simulink model "WindFarm_2023_BaseModel_v2"  (R2019a)
settings: Solver=ode1  StartTime=0.0  StopTime=2  FixedStep=Ts_Power  RelTol=1e-3
PostLoadFcn:
  | %% Init for wind PnO models - global system parameters
  | OVERRIDE_SSN_MEMORY_LIMIT=1;
  | Ts=50e-6;
  | % Ts=50e-10;
  | Ts_Power=Ts;
  | Ts_Control=2*Ts;
  | freq = 50;
  | Fnom=freq;
  | Vac=400e3;
InitFcn:
  | %% Init for wind PnO models - global system parameters
  | OVERRIDE_SSN_MEMORY_LIMIT=1;
  | Ts=50e-6;
  | % Ts=50e-10;
  | Ts_Power=Ts;
  | Ts_Control=2*Ts;
  | freq = 50;
  | Fnom=freq;
  | Vac=220e3;
values from neighbouring files (symbols this model uses):
  C0_Le_1 = C1_Le_1    (= 4.2e-07)    [windfarm_params.m]
  C0_Le_2 = C1_Le_2    (= 4.2e-07)    [windfarm_params.m]
  C0_Le_ON = 0.0084e-6    (= 8.4e-09)    [windfarm_params.m]
  C1_Le_1 = 0.42e-6    (= 4.2e-07)    [windfarm_params.m]
  C1_Le_2 = 0.42e-6    (= 4.2e-07)    [windfarm_params.m]
  C1_Le_ON = 0.0137e-6    (= 1.37e-08)    [windfarm_params.m]
  L0_fLA38a = X0_fLA38a / w    (= 0.00210440713644)    [windfarm_params.m]
  L0_fLB1 = X0_fLB1 / w    (= 0.00146508173004)    [windfarm_params.m]
  L0_fLB2 = X0_fLB2 / w    (= 0.00124721491041)    [windfarm_params.m]
  L0_Le_1 = X0_Le_1 / w    (= 0.00116978883173)    [windfarm_params.m]
  L0_Le_2 = X0_Le_2 / w    (= 0.00116978883173)    [windfarm_params.m]
  L0_Le_ON = 3.1544e-3    (= 0.0031544)    [windfarm_params.m]
  L1_fLA38a = X1_fLA38a / w    (= 0.00070146904548)    [windfarm_params.m]
  L1_fLB1 = X1_fLB1 / w    (= 0.00048836057668)    [windfarm_params.m]
  L1_fLB2 = X1_fLB2 / w    (= 0.000415738303471)    [windfarm_params.m]
  L1_Le_1 = X1_Le_1 / w    (= 0.000389929610575)    [windfarm_params.m]
  L1_Le_2 = X1_Le_2 / w    (= 0.000389929610575)    [windfarm_params.m]
  L1_Le_ON = 0.8467e-3    (= 0.0008467)    [windfarm_params.m]
  length_onshore = 150    [windfarm_params.m]
  length_SM = 60    [windfarm_params.m]
  P_a3_8_1_nom = 450e6    (= 450000000)    [windfarm_params.m]
  P_b_nom = 600e6    (= 600000000)    [windfarm_params.m]
  P_onshore = 500e6    (= 500000000)    [windfarm_params.m]
  R0_fLA38a = R1_fLA38a    (= 0.3514672)    [windfarm_params.m]
  R0_fLB1 = R1_fLB1    (= 0.244686)    [windfarm_params.m]
  R0_fLB2 = R1_fLB2    (= 0.20829138)    [windfarm_params.m]
  R0_Le_1 = R1_Le_1    (= 0.1)    [windfarm_params.m]
  R0_Le_2 = R1_Le_2    (= 0.1)    [windfarm_params.m]
  R0_Le_ON = 0.3030    (= 0.303)    [windfarm_params.m]
  R1_fLA38a = 0.3514672    [windfarm_params.m]
  R1_fLB1 = 0.244686    [windfarm_params.m]
  R1_fLB2 = 0.20829138    [windfarm_params.m]
  R1_Le_1 = 0.1    [windfarm_params.m]
  R1_Le_2 = 0.1    [windfarm_params.m]
  R1_Le_ON = 0.0209    [windfarm_params.m]
  Vgrid = 380e3    (= 380000)    [windfarm_params.m]
  Vnom = 66e3    (= 66000)    [windfarm_params.m]
undefined symbols (not defined in the file or in its folder): D1, D11, Delta, den, DiscIntNeverNeededParam, dx, find_system, gcbh, num, out_Buses, out_WindFarms, sps_rtmsupport
libraries: powerlib x227, simulink x96, powerlib_meascontrol x96, eeSinusoidalMeasurement x63, spsVIMeasurementModel x54, elements x52, simulink_extras x42, eePowerMeasurement x22
(part 13 of 27)

== system WindFarm_2023_BaseModel_v2/SM_WT1/Differential Element 1/Main Protection (Current Differential)/Charging Current Compensation phase C ==
  VA : Inport
  VB : Inport  Port=2
  VC : Inport  Port=3
  " 5" : elements/   fo=Freq  window_size=40  harmonic=[1 2 3 4 5]
  " 6" : elements/   fo=Freq  window_size=40  harmonic=[1 2 3 4 5]
  " 7" : elements/   fo=Freq  window_size=40  harmonic=[1 2 3 4 5]
  *2 : Gain  Gain=2  SaturateOnIntegerOverflow=on  OutDataTypeStr=Inherit: Same as input  ParamDataTypeStr=Inherit: Same as input
  Compensating Current : Sum  SaturateOnIntegerOverflow=on  InputSameDT=on  OutDataTypeStr=Inherit: Same as first input
  Cpg : Gain  Gain=Cpg  SaturateOnIntegerOverflow=on  OutDataTypeStr=Inherit: Same as input  ParamDataTypeStr=Inherit: Same as input
  Cpp : Gain  Gain=Cpp  SaturateOnIntegerOverflow=on  OutDataTypeStr=Inherit: Same as input  ParamDataTypeStr=Inherit: Same as input
  DAB5 : Subsystem  mask(Data Adquisition Board){filter=off, approx=Bessel, order=2, numerator=[], denominator=[], freq=180, resdis=off, vertres=12, xmax=10, winsize=40, G=1.0, fs=Freq*40}
      mask prompts: filter "Disable Analog Filter"; approx "Filter approximation"; numerator "Free expression filter: numerator(descending order of s)"; denominator "Free expression filter: denominator:"; freq "Cut-off frequency"; resdis "Disable Vertical Resolution"; vertres "Vertical Resolution: No. of bits"; xmax "Vertical Resolution: signal range"; winsize "Window size"; G "Gain"; fs "Sampling frequency"
      mask help: Performs analog filtering, signal conditioning and sampling. A single signal is the input, a buffer with the signal samples is the output. The options include analog filter enable/disable switch, type, order and cut-off frequency of the analog filter, conditioning gain, sampling frequency, number of bits, the length of the buffer.
      mask init:
      | dab1
      mask TypeOptions approx: Bessel | Tschebyscheff | Butterworth | free expression
      mask TypeOptions order: 2 | 3 | 4
      mask TypeOptions vertres: 8 | 12 | 16
      mask Display: disp('DAB')
  DAB6 : Subsystem  mask(Data Adquisition Board){filter=off, approx=Bessel, order=2, numerator=[], denominator=[], freq=180, resdis=off, vertres=12, xmax=10, winsize=40, G=1.0, fs=Freq*40}
      mask prompts: filter "Disable Analog Filter"; approx "Filter approximation"; numerator "Free expression filter: numerator(descending order of s)"; denominator "Free expression filter: denominator:"; freq "Cut-off frequency"; resdis "Disable Vertical Resolution"; vertres "Vertical Resolution: No. of bits"; xmax "Vertical Resolution: signal range"; winsize "Window size"; G "Gain"; fs "Sampling frequency"
      mask help: Performs analog filtering, signal conditioning and sampling. A single signal is the input, a buffer with the signal samples is the output. The options include analog filter enable/disable switch, type, order and cut-off frequency of the analog filter, conditioning gain, sampling frequency, number of bits, the length of the buffer.
      mask init:
      | dab1
      mask TypeOptions approx: Bessel | Tschebyscheff | Butterworth | free expression
      mask TypeOptions order: 2 | 3 | 4
      mask TypeOptions vertres: 8 | 12 | 16
      mask Display: disp('DAB')
  DAB7 : Subsystem  mask(Data Adquisition Board){filter=off, approx=Bessel, order=2, numerator=[], denominator=[], freq=180, resdis=off, vertres=12, xmax=10, winsize=40, G=1.0, fs=Freq*40}
      mask prompts: filter "Disable Analog Filter"; approx "Filter approximation"; numerator "Free expression filter: numerator(descending order of s)"; denominator "Free expression filter: denominator:"; freq "Cut-off frequency"; resdis "Disable Vertical Resolution"; vertres "Vertical Resolution: No. of bits"; xmax "Vertical Resolution: signal range"; winsize "Window size"; G "Gain"; fs "Sampling frequency"
      mask help: Performs analog filtering, signal conditioning and sampling. A single signal is the input, a buffer with the signal samples is the output. The options include analog filter enable/disable switch, type, order and cut-off frequency of the analog filter, conditioning gain, sampling frequency, number of bits, the length of the buffer.
      mask init:
      | dab1
      mask TypeOptions approx: Bessel | Tschebyscheff | Butterworth | free expression
      mask TypeOptions order: 2 | 3 | 4
      mask TypeOptions vertres: 8 | 12 | 16
      mask Display: disp('DAB')
  Degrees to Radians1 : simulink_extras/Transformations/Degrees to Radians
  Degrees to Radians2 : simulink_extras/Transformations/Degrees to Radians
  Degrees to Radians3 : simulink_extras/Transformations/Degrees to Radians
  Demux : Demux  Outputs=2
  Demux1 : Demux  Outputs=2
  Demux2 : Demux  Outputs=2
  Derivative : Derivative
  Derivative1 : Derivative
  Derivative2 : Derivative
  Magnitude-Angle to Complex : MagnitudeAngleToComplex
  Magnitude-Angle to Complex1 : MagnitudeAngleToComplex
  Magnitude-Angle to Complex2 : MagnitudeAngleToComplex
  Mux : Mux  Inputs=12
  Terminator : Terminator
  sum : Sum  Inputs=+--  SaturateOnIntegerOverflow=on  InputSameDT=on  OutDataTypeStr=Inherit: Same as first input
  Icomp : Outport  VectorParamsAs1DForOutWhenUnconnected=on
  wires:
  VA/1 -> Derivative2/1
  VC/1 -> Derivative/1
  " 5"/1 -> Demux2/1
  Demux1/2 -> Degrees to Radians2/1
  Demux1/1 -> Magnitude-Angle to Complex1/1
  " 7"/1 -> Demux/1
  Derivative1/1 -> DAB6/1(a)
  DAB6/1(d) -> " 6"/1
  " 6"/1 -> Demux1/1
  VB/1 -> Derivative1/1
  Mux/1 -> Terminator/1
  " 5"/5 -> Mux/4
  Derivative/1 -> DAB5/1(a)
  DAB5/1(d) -> " 5"/1
  Cpg/1 -> Compensating Current/1
  " 5"/2 -> Mux/1
  " 5"/3 -> Mux/2
  " 5"/4 -> Mux/3
  sum/1 -> Cpp/1
  Compensating Current/1 -> Icomp/1
  *2/1 -> sum/1
  Cpp/1 -> Compensating Current/2
  Derivative2/1 -> DAB7/1(a)
  DAB7/1(d) -> " 7"/1
  " 7"/2 -> Mux/9
  " 7"/3 -> Mux/10
  " 7"/4 -> Mux/11
  " 7"/5 -> Mux/12
  " 6"/2 -> Mux/5
  " 6"/3 -> Mux/6
  " 6"/4 -> Mux/7
  " 6"/5 -> Mux/8
  Demux2/1 -> Magnitude-Angle to Complex/1
  Magnitude-Angle to Complex/1 -> *2/1, Cpg/1
  Magnitude-Angle to Complex1/1 -> sum/2
  Demux/1 -> Magnitude-Angle to Complex2/1
  Magnitude-Angle to Complex2/1 -> sum/3
  Demux/2 -> Degrees to Radians1/1
  Degrees to Radians1/1 -> Magnitude-Angle to Complex2/2
  Degrees to Radians2/1 -> Magnitude-Angle to Complex1/2
  Demux2/2 -> Degrees to Radians3/1
  Degrees to Radians3/1 -> Magnitude-Angle to Complex/2

== system WindFarm_2023_BaseModel_v2/SM_WT1/Differential Element 1/Main Protection (Current Differential)/Current Differential Protection for Phase A ==
  Ilocal : Inport
  Iremote : Inport  Port=2
  Icomp : Inport  Port=3
  " " : elements/   fo=Freq  window_size=40  harmonic=[1 2 3 4 5]
  " 1" : elements/   fo=Freq  window_size=40  harmonic=[1 2 3 4 5]
  Comparing Current at Master Station : Sum  Inputs=+-  SaturateOnIntegerOverflow=on  InputSameDT=on  OutDataTypeStr=Inherit: Same as first input
  Comparision Scheme : Subsystem
  DAB4 : Subsystem  mask(Data Adquisition Board){filter=off, approx=Bessel, order=2, numerator=[], denominator=[], freq=180, resdis=off, vertres=12, xmax=10, winsize=40, G=1.0, fs=Freq*40}
      mask prompts: filter "Disable Analog Filter"; approx "Filter approximation"; numerator "Free expression filter: numerator(descending order of s)"; denominator "Free expression filter: denominator:"; freq "Cut-off frequency"; resdis "Disable Vertical Resolution"; vertres "Vertical Resolution: No. of bits"; xmax "Vertical Resolution: signal range"; winsize "Window size"; G "Gain"; fs "Sampling frequency"
      mask help: Performs analog filtering, signal conditioning and sampling. A single signal is the input, a buffer with the signal samples is the output. The options include analog filter enable/disable switch, type, order and cut-off frequency of the analog filter, conditioning gain, sampling frequency, number of bits, the length of the buffer.
      mask init:
      | dab1
      mask TypeOptions approx: Bessel | Tschebyscheff | Butterworth | free expression
      mask TypeOptions order: 2 | 3 | 4
      mask TypeOptions vertres: 8 | 12 | 16
      mask Display: disp('DAB')
  DAB8 : Subsystem  mask(Data Adquisition Board){filter=off, approx=Bessel, order=2, numerator=[], denominator=[], freq=180, resdis=off, vertres=12, xmax=10, winsize=40, G=1.0, fs=Freq*40}
      mask prompts: filter "Disable Analog Filter"; approx "Filter approximation"; numerator "Free expression filter: numerator(descending order of s)"; denominator "Free expression filter: denominator:"; freq "Cut-off frequency"; resdis "Disable Vertical Resolution"; vertres "Vertical Resolution: No. of bits"; xmax "Vertical Resolution: signal range"; winsize "Window size"; G "Gain"; fs "Sampling frequency"
      mask help: Performs analog filtering, signal conditioning and sampling. A single signal is the input, a buffer with the signal samples is the output. The options include analog filter enable/disable switch, type, order and cut-off frequency of the analog filter, conditioning gain, sampling frequency, number of bits, the length of the buffer.
      mask init:
      | dab1
      mask TypeOptions approx: Bessel | Tschebyscheff | Butterworth | free expression
      mask TypeOptions order: 2 | 3 | 4
      mask TypeOptions vertres: 8 | 12 | 16
      mask Display: disp('DAB')
  Degrees to Radians : simulink_extras/Transformations/Degrees to Radians
  Degrees to Radians1 : simulink_extras/Transformations/Degrees to Radians
  Demux1 : Demux  Outputs=2
  Demux2 : Demux  Outputs=2
  Gain : Gain  SaturateOnIntegerOverflow=on  OutDataTypeStr=Inherit: Same as input  ParamDataTypeStr=Inherit: Same as input
  Gain1 : Gain  SaturateOnIntegerOverflow=on  OutDataTypeStr=Inherit: Same as input  ParamDataTypeStr=Inherit: Same as input
  Magnitude-Angle to Complex : MagnitudeAngleToComplex
  Magnitude-Angle to Complex1 : MagnitudeAngleToComplex
  Mux1 : Mux
  Mux2 : Mux
  Terminator1 : Terminator
  Terminator2 : Terminator
  Trip : Outport  InitialOutput=0  VectorParamsAs1DForOutWhenUnconnected=on
  wires:
  Gain1/1 -> Comparing Current at Master Station/2
  " 1"/2 -> Mux2/1
  " 1"/4 -> Mux2/3
  " 1"/3 -> Mux2/2
  Mux2/1 -> Terminator2/1
  Gain/1 -> DAB8/1(a)
  Iremote/1 -> Gain/1
  " 1"/1 -> Demux2/1
  DAB8/1(d) -> " 1"/1
  Magnitude-Angle to Complex1/1 -> Comparision Scheme/2(I_Master)
  Demux2/2 -> Degrees to Radians/1
  Degrees to Radians/1 -> Magnitude-Angle to Complex1/2
  Demux2/1 -> Magnitude-Angle to Complex1/1
  " "/5 -> Mux1/4
  " "/4 -> Mux1/3
  " "/3 -> Mux1/2
  " "/2 -> Mux1/1
  Mux1/1 -> Terminator1/1
  " "/1 -> Demux1/1
  Comparision Scheme/1(Pickup) -> Trip/1
  DAB4/1(d) -> " "/1
  Ilocal/1 -> DAB4/1(a)
  Magnitude-Angle to Complex/1 -> Comparing Current at Master Station/1
  Icomp/1 -> Gain1/1
  Demux1/2 -> Degrees to Radians1/1
  Degrees to Radians1/1 -> Magnitude-Angle to Complex/2
  Comparing Current at Master Station/1 -> Comparision Scheme/1(I_Slave)
  " 1"/5 -> Mux2/4
  Demux1/1 -> Magnitude-Angle to Complex/1

== system WindFarm_2023_BaseModel_v2/SM_WT1/Differential Element 1/Main Protection (Current Differential)/Current Differential Protection for Phase B ==
  Ilocal : Inport
  Iremote : Inport  Port=2
  Icomp : Inport  Port=3
  " " : elements/   fo=Freq  window_size=40  harmonic=[1 2 3 4 5]
  " 1" : elements/   fo=Freq  window_size=40  harmonic=[1 2 3 4 5]
  Comparing Current at Master Station : Sum  Inputs=+-  SaturateOnIntegerOverflow=on  InputSameDT=on  OutDataTypeStr=Inherit: Same as first input
  Comparision Scheme : Subsystem
  DAB4 : Subsystem  mask(Data Adquisition Board){filter=off, approx=Bessel, order=2, numerator=[], denominator=[], freq=180, resdis=off, vertres=12, xmax=10, winsize=40, G=1.0, fs=Freq*40}
      mask prompts: filter "Disable Analog Filter"; approx "Filter approximation"; numerator "Free expression filter: numerator(descending order of s)"; denominator "Free expression filter: denominator:"; freq "Cut-off frequency"; resdis "Disable Vertical Resolution"; vertres "Vertical Resolution: No. of bits"; xmax "Vertical Resolution: signal range"; winsize "Window size"; G "Gain"; fs "Sampling frequency"
      mask help: Performs analog filtering, signal conditioning and sampling. A single signal is the input, a buffer with the signal samples is the output. The options include analog filter enable/disable switch, type, order and cut-off frequency of the analog filter, conditioning gain, sampling frequency, number of bits, the length of the buffer.
      mask init:
      | dab1
      mask TypeOptions approx: Bessel | Tschebyscheff | Butterworth | free expression
      mask TypeOptions order: 2 | 3 | 4
      mask TypeOptions vertres: 8 | 12 | 16
      mask Display: disp('DAB')
  DAB8 : Subsystem  mask(Data Adquisition Board){filter=off, approx=Bessel, order=2, numerator=[], denominator=[], freq=180, resdis=off, vertres=12, xmax=10, winsize=40, G=1.0, fs=Freq*40}
      mask prompts: filter "Disable Analog Filter"; approx "Filter approximation"; numerator "Free expression filter: numerator(descending order of s)"; denominator "Free expression filter: denominator:"; freq "Cut-off frequency"; resdis "Disable Vertical Resolution"; vertres "Vertical Resolution: No. of bits"; xmax "Vertical Resolution: signal range"; winsize "Window size"; G "Gain"; fs "Sampling frequency"
      mask help: Performs analog filtering, signal conditioning and sampling. A single signal is the input, a buffer with the signal samples is the output. The options include analog filter enable/disable switch, type, order and cut-off frequency of the analog filter, conditioning gain, sampling frequency, number of bits, the length of the buffer.
      mask init:
      | dab1
      mask TypeOptions approx: Bessel | Tschebyscheff | Butterworth | free expression
      mask TypeOptions order: 2 | 3 | 4
      mask TypeOptions vertres: 8 | 12 | 16
      mask Display: disp('DAB')
  Degrees to Radians : simulink_extras/Transformations/Degrees to Radians
  Degrees to Radians1 : simulink_extras/Transformations/Degrees to Radians
  Demux1 : Demux  Outputs=2
  Demux2 : Demux  Outputs=2
  Gain : Gain  SaturateOnIntegerOverflow=on  OutDataTypeStr=Inherit: Same as input  ParamDataTypeStr=Inherit: Same as input
  Gain1 : Gain  SaturateOnIntegerOverflow=on  OutDataTypeStr=Inherit: Same as input  ParamDataTypeStr=Inherit: Same as input
  Magnitude-Angle to Complex : MagnitudeAngleToComplex
  Magnitude-Angle to Complex1 : MagnitudeAngleToComplex
  Mux1 : Mux
  Mux2 : Mux
  Terminator1 : Terminator
  Terminator2 : Terminator
  Trip : Outport  InitialOutput=0  VectorParamsAs1DForOutWhenUnconnected=on
  wires:
  Gain1/1 -> Comparing Current at Master Station/2
  Demux1/1 -> Magnitude-Angle to Complex/1
  " 1"/5 -> Mux2/4
  Comparing Current at Master Station/1 -> Comparision Scheme/1(I_Slave)
  Degrees to Radians1/1 -> Magnitude-Angle to Complex/2
  Demux1/2 -> Degrees to Radians1/1
  Icomp/1 -> Gain1/1
  Magnitude-Angle to Complex/1 -> Comparing Current at Master Station/1
  Ilocal/1 -> DAB4/1(a)
  DAB4/1(d) -> " "/1
  Comparision Scheme/1(Pickup) -> Trip/1
  " "/1 -> Demux1/1
  Mux1/1 -> Terminator1/1
  " "/2 -> Mux1/1
  " "/3 -> Mux1/2
  " "/4 -> Mux1/3
  " "/5 -> Mux1/4
  Demux2/1 -> Magnitude-Angle to Complex1/1
  Degrees to Radians/1 -> Magnitude-Angle to Complex1/2
  Demux2/2 -> Degrees to Radians/1
  Magnitude-Angle to Complex1/1 -> Comparision Scheme/2(I_Master)
  DAB8/1(d) -> " 1"/1
  " 1"/1 -> Demux2/1
  Iremote/1 -> Gain/1
  Gain/1 -> DAB8/1(a)
  Mux2/1 -> Terminator2/1
  " 1"/3 -> Mux2/2
  " 1"/4 -> Mux2/3
  " 1"/2 -> Mux2/1

== system WindFarm_2023_BaseModel_v2/SM_WT1/Differential Element 1/Main Protection (Current Differential)/Current Differential Protection for Phase C ==
  Ilocal : Inport
  Iremote : Inport  Port=2
  Icomp : Inport  Port=3
  " " : elements/   fo=Freq  window_size=40  harmonic=[1 2 3 4 5]
  " 1" : elements/   fo=Freq  window_size=40  harmonic=[1 2 3 4 5]
  Comparing Current at Master Station : Sum  Inputs=+-  SaturateOnIntegerOverflow=on  InputSameDT=on  OutDataTypeStr=Inherit: Same as first input
  Comparision Scheme : Subsystem
  DAB4 : Subsystem  mask(Data Adquisition Board){filter=off, approx=Bessel, order=2, numerator=[], denominator=[], freq=180, resdis=off, vertres=12, xmax=10, winsize=40, G=1.0, fs=Freq*40}
      mask prompts: filter "Disable Analog Filter"; approx "Filter approximation"; numerator "Free expression filter: numerator(descending order of s)"; denominator "Free expression filter: denominator:"; freq "Cut-off frequency"; resdis "Disable Vertical Resolution"; vertres "Vertical Resolution: No. of bits"; xmax "Vertical Resolution: signal range"; winsize "Window size"; G "Gain"; fs "Sampling frequency"
      mask help: Performs analog filtering, signal conditioning and sampling. A single signal is the input, a buffer with the signal samples is the output. The options include analog filter enable/disable switch, type, order and cut-off frequency of the analog filter, conditioning gain, sampling frequency, number of bits, the length of the buffer.
      mask init:
      | dab1
      mask TypeOptions approx: Bessel | Tschebyscheff | Butterworth | free expression
      mask TypeOptions order: 2 | 3 | 4
      mask TypeOptions vertres: 8 | 12 | 16
      mask Display: disp('DAB')
  DAB8 : Subsystem  mask(Data Adquisition Board){filter=off, approx=Bessel, order=2, numerator=[], denominator=[], freq=180, resdis=off, vertres=12, xmax=10, winsize=40, G=1.0, fs=Freq*40}
      mask prompts: filter "Disable Analog Filter"; approx "Filter approximation"; numerator "Free expression filter: numerator(descending order of s)"; denominator "Free expression filter: denominator:"; freq "Cut-off frequency"; resdis "Disable Vertical Resolution"; vertres "Vertical Resolution: No. of bits"; xmax "Vertical Resolution: signal range"; winsize "Window size"; G "Gain"; fs "Sampling frequency"
      mask help: Performs analog filtering, signal conditioning and sampling. A single signal is the input, a buffer with the signal samples is the output. The options include analog filter enable/disable switch, type, order and cut-off frequency of the analog filter, conditioning gain, sampling frequency, number of bits, the length of the buffer.
      mask init:
      | dab1
      mask TypeOptions approx: Bessel | Tschebyscheff | Butterworth | free expression
      mask TypeOptions order: 2 | 3 | 4
      mask TypeOptions vertres: 8 | 12 | 16
      mask Display: disp('DAB')
  Degrees to Radians : simulink_extras/Transformations/Degrees to Radians
  Degrees to Radians1 : simulink_extras/Transformations/Degrees to Radians
  Demux1 : Demux  Outputs=2
  Demux2 : Demux  Outputs=2
  Gain : Gain  SaturateOnIntegerOverflow=on  OutDataTypeStr=Inherit: Same as input  ParamDataTypeStr=Inherit: Same as input
  Gain1 : Gain  SaturateOnIntegerOverflow=on  OutDataTypeStr=Inherit: Same as input  ParamDataTypeStr=Inherit: Same as input
  Magnitude-Angle to Complex : MagnitudeAngleToComplex
  Magnitude-Angle to Complex1 : MagnitudeAngleToComplex
  Mux1 : Mux
  Mux2 : Mux
  Terminator1 : Terminator
  Terminator2 : Terminator
  Trip : Outport  InitialOutput=0  VectorParamsAs1DForOutWhenUnconnected=on
  wires:
  Gain1/1 -> Comparing Current at Master Station/2
  " 1"/2 -> Mux2/1
  " 1"/4 -> Mux2/3
  " 1"/3 -> Mux2/2
  Mux2/1 -> Terminator2/1
  Gain/1 -> DAB8/1(a)
  Iremote/1 -> Gain/1
  " 1"/1 -> Demux2/1
  DAB8/1(d) -> " 1"/1
  Magnitude-Angle to Complex1/1 -> Comparision Scheme/2(I_Master)
  Demux2/2 -> Degrees to Radians/1
  Degrees to Radians/1 -> Magnitude-Angle to Complex1/2
  Demux2/1 -> Magnitude-Angle to Complex1/1
  " "/5 -> Mux1/4
  " "/4 -> Mux1/3
  " "/3 -> Mux1/2
  " "/2 -> Mux1/1
  Mux1/1 -> Terminator1/1
  " "/1 -> Demux1/1
  Comparision Scheme/1(Pickup) -> Trip/1
  DAB4/1(d) -> " "/1
  Ilocal/1 -> DAB4/1(a)
  Magnitude-Angle to Complex/1 -> Comparing Current at Master Station/1
  Icomp/1 -> Gain1/1
  Demux1/2 -> Degrees to Radians1/1
  Degrees to Radians1/1 -> Magnitude-Angle to Complex/2
  Comparing Current at Master Station/1 -> Comparision Scheme/1(I_Slave)
  " 1"/5 -> Mux2/4
  Demux1/1 -> Magnitude-Angle to Complex/1

== system WindFarm_2023_BaseModel_v2/SM_WT1/Differential Element 2/Main Protection (Current Differential)/Charging Current Compensation phase A ==
  VA : Inport
  VB : Inport  Port=2
  VC : Inport  Port=3
  " 5" : elements/   fo=Freq  window_size=40  harmonic=[1 2 3 4 5]
  " 6" : elements/   fo=Freq  window_size=40  harmonic=[1 2 3 4 5]
  " 7" : elements/   fo=Freq  window_size=40  harmonic=[1 2 3 4 5]
  *2 : Gain  Gain=2  SaturateOnIntegerOverflow=on  OutDataTypeStr=Inherit: Same as input  ParamDataTypeStr=Inherit: Same as input
  Compensating Current : Sum  SaturateOnIntegerOverflow=on  InputSameDT=on  OutDataTypeStr=Inherit: Same as first input
  Cpg : Gain  Gain=Cpg  SaturateOnIntegerOverflow=on  OutDataTypeStr=Inherit: Same as input  ParamDataTypeStr=Inherit: Same as input
  Cpp : Gain  Gain=Cpp  SaturateOnIntegerOverflow=on  OutDataTypeStr=Inherit: Same as input  ParamDataTypeStr=Inherit: Same as input
  DAB5 : Subsystem  mask(Data Adquisition Board){filter=off, approx=Bessel, order=2, numerator=[], denominator=[], freq=180, resdis=off, vertres=12, xmax=10, winsize=40, G=1.0, fs=Freq*40}
      mask prompts: filter "Disable Analog Filter"; approx "Filter approximation"; numerator "Free expression filter: numerator(descending order of s)"; denominator "Free expression filter: denominator:"; freq "Cut-off frequency"; resdis "Disable Vertical Resolution"; vertres "Vertical Resolution: No. of bits"; xmax "Vertical Resolution: signal range"; winsize "Window size"; G "Gain"; fs "Sampling frequency"
      mask help: Performs analog filtering, signal conditioning and sampling. A single signal is the input, a buffer with the signal samples is the output. The options include analog filter enable/disable switch, type, order and cut-off frequency of the analog filter, conditioning gain, sampling frequency, number of bits, the length of the buffer.
      mask init:
      | dab1
      mask TypeOptions approx: Bessel | Tschebyscheff | Butterworth | free expression
      mask TypeOptions order: 2 | 3 | 4
      mask TypeOptions vertres: 8 | 12 | 16
      mask Display: disp('DAB')
  DAB6 : Subsystem  mask(Data Adquisition Board){filter=off, approx=Bessel, order=2, numerator=[], denominator=[], freq=180, resdis=off, vertres=12, xmax=10, winsize=40, G=1.0, fs=Freq*40}
      mask prompts: filter "Disable Analog Filter"; approx "Filter approximation"; numerator "Free expression filter: numerator(descending order of s)"; denominator "Free expression filter: denominator:"; freq "Cut-off frequency"; resdis "Disable Vertical Resolution"; vertres "Vertical Resolution: No. of bits"; xmax "Vertical Resolution: signal range"; winsize "Window size"; G "Gain"; fs "Sampling frequency"
      mask help: Performs analog filtering, signal conditioning and sampling. A single signal is the input, a buffer with the signal samples is the output. The options include analog filter enable/disable switch, type, order and cut-off frequency of the analog filter, conditioning gain, sampling frequency, number of bits, the length of the buffer.
      mask init:
      | dab1
      mask TypeOptions approx: Bessel | Tschebyscheff | Butterworth | free expression
      mask TypeOptions order: 2 | 3 | 4
      mask TypeOptions vertres: 8 | 12 | 16
      mask Display: disp('DAB')
  DAB7 : Subsystem  mask(Data Adquisition Board){filter=off, approx=Bessel, order=2, numerator=[], denominator=[], freq=180, resdis=off, vertres=12, xmax=10, winsize=40, G=1.0, fs=Freq*40}
      mask prompts: filter "Disable Analog Filter"; approx "Filter approximation"; numerator "Free expression filter: numerator(descending order of s)"; denominator "Free expression filter: denominator:"; freq "Cut-off frequency"; resdis "Disable Vertical Resolution"; vertres "Vertical Resolution: No. of bits"; xmax "Vertical Resolution: signal range"; winsize "Window size"; G "Gain"; fs "Sampling frequency"
      mask help: Performs analog filtering, signal conditioning and sampling. A single signal is the input, a buffer with the signal samples is the output. The options include analog filter enable/disable switch, type, order and cut-off frequency of the analog filter, conditioning gain, sampling frequency, number of bits, the length of the buffer.
      mask init:
      | dab1
      mask TypeOptions approx: Bessel | Tschebyscheff | Butterworth | free expression
      mask TypeOptions order: 2 | 3 | 4
      mask TypeOptions vertres: 8 | 12 | 16
      mask Display: disp('DAB')
  Degrees to Radians1 : simulink_extras/Transformations/Degrees to Radians
  Degrees to Radians2 : simulink_extras/Transformations/Degrees to Radians
  Degrees to Radians3 : simulink_extras/Transformations/Degrees to Radians
  Demux : Demux  Outputs=2
  Demux1 : Demux  Outputs=2
  Demux2 : Demux  Outputs=2
  Derivative : Derivative
  Derivative1 : Derivative
  Derivative2 : Derivative
  Magnitude-Angle to Complex : MagnitudeAngleToComplex
  Magnitude-Angle to Complex1 : MagnitudeAngleToComplex
  Magnitude-Angle to Complex2 : MagnitudeAngleToComplex
  Mux : Mux  Inputs=12
  Terminator : Terminator
  sum : Sum  Inputs=+--  SaturateOnIntegerOverflow=on  InputSameDT=on  OutDataTypeStr=Inherit: Same as first input
  Icomp : Outport  VectorParamsAs1DForOutWhenUnconnected=on
  wires:
  " 5"/1 -> Demux2/1
  Demux1/2 -> Degrees to Radians2/1
  Demux1/1 -> Magnitude-Angle to Complex1/1
  " 7"/1 -> Demux/1
  Derivative1/1 -> DAB6/1(a)
  DAB6/1(d) -> " 6"/1
  " 6"/1 -> Demux1/1
  VB/1 -> Derivative1/1
  Mux/1 -> Terminator/1
  " 5"/5 -> Mux/4
  Derivative/1 -> DAB5/1(a)
  DAB5/1(d) -> " 5"/1
  Cpg/1 -> Compensating Current/1
  VA/1 -> Derivative/1
  " 5"/2 -> Mux/1
  " 5"/3 -> Mux/2
  " 5"/4 -> Mux/3
  sum/1 -> Cpp/1
  Compensating Current/1 -> Icomp/1
  *2/1 -> sum/1
  Cpp/1 -> Compensating Current/2
  Derivative2/1 -> DAB7/1(a)
  DAB7/1(d) -> " 7"/1
  VC/1 -> Derivative2/1
  " 7"/2 -> Mux/9
  " 7"/3 -> Mux/10
  " 7"/4 -> Mux/11
  " 7"/5 -> Mux/12
  " 6"/2 -> Mux/5
  " 6"/3 -> Mux/6
  " 6"/4 -> Mux/7
  " 6"/5 -> Mux/8
  Demux2/1 -> Magnitude-Angle to Complex/1
  Magnitude-Angle to Complex/1 -> *2/1, Cpg/1
  Magnitude-Angle to Complex1/1 -> sum/2
  Demux/1 -> Magnitude-Angle to Complex2/1
  Magnitude-Angle to Complex2/1 -> sum/3
  Demux/2 -> Degrees to Radians1/1
  Degrees to Radians1/1 -> Magnitude-Angle to Complex2/2
  Degrees to Radians2/1 -> Magnitude-Angle to Complex1/2
  Demux2/2 -> Degrees to Radians3/1
  Degrees to Radians3/1 -> Magnitude-Angle to Complex/2

== system WindFarm_2023_BaseModel_v2/SM_WT1/Differential Element 2/Main Protection (Current Differential)/Charging Current Compensation phase B ==
  VA : Inport
  VB : Inport  Port=2
  VC : Inport  Port=3
  " 5" : elements/   fo=Freq  window_size=40  harmonic=[1 2 3 4 5]
  " 6" : elements/   fo=Freq  window_size=40  harmonic=[1 2 3 4 5]
  " 7" : elements/   fo=Freq  window_size=40  harmonic=[1 2 3 4 5]
  *2 : Gain  Gain=2  SaturateOnIntegerOverflow=on  OutDataTypeStr=Inherit: Same as input  ParamDataTypeStr=Inherit: Same as input
  Compensating Current : Sum  SaturateOnIntegerOverflow=on  InputSameDT=on  OutDataTypeStr=Inherit: Same as first input
  Cpg : Gain  Gain=Cpg  SaturateOnIntegerOverflow=on  OutDataTypeStr=Inherit: Same as input  ParamDataTypeStr=Inherit: Same as input
  Cpp : Gain  Gain=Cpp  SaturateOnIntegerOverflow=on  OutDataTypeStr=Inherit: Same as input  ParamDataTypeStr=Inherit: Same as input
  DAB5 : Subsystem  mask(Data Adquisition Board){filter=off, approx=Bessel, order=2, numerator=[], denominator=[], freq=180, resdis=off, vertres=12, xmax=10, winsize=40, G=1.0, fs=Freq*40}
      mask prompts: filter "Disable Analog Filter"; approx "Filter approximation"; numerator "Free expression filter: numerator(descending order of s)"; denominator "Free expression filter: denominator:"; freq "Cut-off frequency"; resdis "Disable Vertical Resolution"; vertres "Vertical Resolution: No. of bits"; xmax "Vertical Resolution: signal range"; winsize "Window size"; G "Gain"; fs "Sampling frequency"
      mask help: Performs analog filtering, signal conditioning and sampling. A single signal is the input, a buffer with the signal samples is the output. The options include analog filter enable/disable switch, type, order and cut-off frequency of the analog filter, conditioning gain, sampling frequency, number of bits, the length of the buffer.
      mask init:
      | dab1
      mask TypeOptions approx: Bessel | Tschebyscheff | Butterworth | free expression
      mask TypeOptions order: 2 | 3 | 4
      mask TypeOptions vertres: 8 | 12 | 16
      mask Display: disp('DAB')
  DAB6 : Subsystem  mask(Data Adquisition Board){filter=off, approx=Bessel, order=2, numerator=[], denominator=[], freq=180, resdis=off, vertres=12, xmax=10, winsize=40, G=1.0, fs=Freq*40}
      mask prompts: filter "Disable Analog Filter"; approx "Filter approximation"; numerator "Free expression filter: numerator(descending order of s)"; denominator "Free expression filter: denominator:"; freq "Cut-off frequency"; resdis "Disable Vertical Resolution"; vertres "Vertical Resolution: No. of bits"; xmax "Vertical Resolution: signal range"; winsize "Window size"; G "Gain"; fs "Sampling frequency"
      mask help: Performs analog filtering, signal conditioning and sampling. A single signal is the input, a buffer with the signal samples is the output. The options include analog filter enable/disable switch, type, order and cut-off frequency of the analog filter, conditioning gain, sampling frequency, number of bits, the length of the buffer.
      mask init:
      | dab1
      mask TypeOptions approx: Bessel | Tschebyscheff | Butterworth | free expression
      mask TypeOptions order: 2 | 3 | 4
      mask TypeOptions vertres: 8 | 12 | 16
      mask Display: disp('DAB')
  DAB7 : Subsystem  mask(Data Adquisition Board){filter=off, approx=Bessel, order=2, numerator=[], denominator=[], freq=180, resdis=off, vertres=12, xmax=10, winsize=40, G=1.0, fs=Freq*40}
      mask prompts: filter "Disable Analog Filter"; approx "Filter approximation"; numerator "Free expression filter: numerator(descending order of s)"; denominator "Free expression filter: denominator:"; freq "Cut-off frequency"; resdis "Disable Vertical Resolution"; vertres "Vertical Resolution: No. of bits"; xmax "Vertical Resolution: signal range"; winsize "Window size"; G "Gain"; fs "Sampling frequency"
      mask help: Performs analog filtering, signal conditioning and sampling. A single signal is the input, a buffer with the signal samples is the output. The options include analog filter enable/disable switch, type, order and cut-off frequency of the analog filter, conditioning gain, sampling frequency, number of bits, the length of the buffer.
      mask init:
      | dab1
      mask TypeOptions approx: Bessel | Tschebyscheff | Butterworth | free expression
      mask TypeOptions order: 2 | 3 | 4
      mask TypeOptions vertres: 8 | 12 | 16
      mask Display: disp('DAB')
  Degrees to Radians1 : simulink_extras/Transformations/Degrees to Radians
  Degrees to Radians2 : simulink_extras/Transformations/Degrees to Radians
  Degrees to Radians3 : simulink_extras/Transformations/Degrees to Radians
  Demux : Demux  Outputs=2
  Demux1 : Demux  Outputs=2
  Demux2 : Demux  Outputs=2
  Derivative : Derivative
  Derivative1 : Derivative
  Derivative2 : Derivative
  Magnitude-Angle to Complex : MagnitudeAngleToComplex
  Magnitude-Angle to Complex1 : MagnitudeAngleToComplex
  Magnitude-Angle to Complex2 : MagnitudeAngleToComplex
  Mux : Mux  Inputs=12
  Terminator : Terminator
  sum : Sum  Inputs=+--  SaturateOnIntegerOverflow=on  InputSameDT=on  OutDataTypeStr=Inherit: Same as first input
  Icomp : Outport  VectorParamsAs1DForOutWhenUnconnected=on
  wires:
  VA/1 -> Derivative1/1
  VB/1 -> Derivative/1
  " 5"/1 -> Demux2/1
  Demux1/2 -> Degrees to Radians2/1
  Demux1/1 -> Magnitude-Angle to Complex1/1
  " 7"/1 -> Demux/1
  Derivative1/1 -> DAB6/1(a)
  DAB6/1(d) -> " 6"/1
  " 6"/1 -> Demux1/1
  Mux/1 -> Terminator/1
  " 5"/5 -> Mux/4
  Derivative/1 -> DAB5/1(a)
  DAB5/1(d) -> " 5"/1
  Cpg/1 -> Compensating Current/1
  " 5"/2 -> Mux/1
  " 5"/3 -> Mux/2
  " 5"/4 -> Mux/3
  sum/1 -> Cpp/1
  Compensating Current/1 -> Icomp/1
  *2/1 -> sum/1
  Cpp/1 -> Compensating Current/2
  Derivative2/1 -> DAB7/1(a)
  DAB7/1(d) -> " 7"/1
  VC/1 -> Derivative2/1
  " 7"/2 -> Mux/9
  " 7"/3 -> Mux/10
  " 7"/4 -> Mux/11
  " 7"/5 -> Mux/12
  " 6"/2 -> Mux/5
  " 6"/3 -> Mux/6
  " 6"/4 -> Mux/7
  " 6"/5 -> Mux/8
  Demux2/1 -> Magnitude-Angle to Complex/1
  Magnitude-Angle to Complex/1 -> *2/1, Cpg/1
  Magnitude-Angle to Complex1/1 -> sum/2
  Demux/1 -> Magnitude-Angle to Complex2/1
  Magnitude-Angle to Complex2/1 -> sum/3
  Demux/2 -> Degrees to Radians1/1
  Degrees to Radians1/1 -> Magnitude-Angle to Complex2/2
  Degrees to Radians2/1 -> Magnitude-Angle to Complex1/2
  Demux2/2 -> Degrees to Radians3/1
  Degrees to Radians3/1 -> Magnitude-Angle to Complex/2

== system WindFarm_2023_BaseModel_v2/SM_WT1/Differential Element 2/Main Protection (Current Differential)/Charging Current Compensation phase C ==
  VA : Inport
  VB : Inport  Port=2
  VC : Inport  Port=3
  " 5" : elements/   fo=Freq  window_size=40  harmonic=[1 2 3 4 5]
  " 6" : elements/   fo=Freq  window_size=40  harmonic=[1 2 3 4 5]
  " 7" : elements/   fo=Freq  window_size=40  harmonic=[1 2 3 4 5]
  *2 : Gain  Gain=2  SaturateOnIntegerOverflow=on  OutDataTypeStr=Inherit: Same as input  ParamDataTypeStr=Inherit: Same as input
  Compensating Current : Sum  SaturateOnIntegerOverflow=on  InputSameDT=on  OutDataTypeStr=Inherit: Same as first input
  Cpg : Gain  Gain=Cpg  SaturateOnIntegerOverflow=on  OutDataTypeStr=Inherit: Same as input  ParamDataTypeStr=Inherit: Same as input
  Cpp : Gain  Gain=Cpp  SaturateOnIntegerOverflow=on  OutDataTypeStr=Inherit: Same as input  ParamDataTypeStr=Inherit: Same as input
  DAB5 : Subsystem  mask(Data Adquisition Board){filter=off, approx=Bessel, order=2, numerator=[], denominator=[], freq=180, resdis=off, vertres=12, xmax=10, winsize=40, G=1.0, fs=Freq*40}
      mask prompts: filter "Disable Analog Filter"; approx "Filter approximation"; numerator "Free expression filter: numerator(descending order of s)"; denominator "Free expression filter: denominator:"; freq "Cut-off frequency"; resdis "Disable Vertical Resolution"; vertres "Vertical Resolution: No. of bits"; xmax "Vertical Resolution: signal range"; winsize "Window size"; G "Gain"; fs "Sampling frequency"
      mask help: Performs analog filtering, signal conditioning and sampling. A single signal is the input, a buffer with the signal samples is the output. The options include analog filter enable/disable switch, type, order and cut-off frequency of the analog filter, conditioning gain, sampling frequency, number of bits, the length of the buffer.
      mask init:
      | dab1
      mask TypeOptions approx: Bessel | Tschebyscheff | Butterworth | free expression
      mask TypeOptions order: 2 | 3 | 4
      mask TypeOptions vertres: 8 | 12 | 16
      mask Display: disp('DAB')
  DAB6 : Subsystem  mask(Data Adquisition Board){filter=off, approx=Bessel, order=2, numerator=[], denominator=[], freq=180, resdis=off, vertres=12, xmax=10, winsize=40, G=1.0, fs=Freq*40}
      mask prompts: filter "Disable Analog Filter"; approx "Filter approximation"; numerator "Free expression filter: numerator(descending order of s)"; denominator "Free expression filter: denominator:"; freq "Cut-off frequency"; resdis "Disable Vertical Resolution"; vertres "Vertical Resolution: No. of bits"; xmax "Vertical Resolution: signal range"; winsize "Window size"; G "Gain"; fs "Sampling frequency"
      mask help: Performs analog filtering, signal conditioning and sampling. A single signal is the input, a buffer with the signal samples is the output. The options include analog filter enable/disable switch, type, order and cut-off frequency of the analog filter, conditioning gain, sampling frequency, number of bits, the length of the buffer.
      mask init:
      | dab1
      mask TypeOptions approx: Bessel | Tschebyscheff | Butterworth | free expression
      mask TypeOptions order: 2 | 3 | 4
      mask TypeOptions vertres: 8 | 12 | 16
      mask Display: disp('DAB')
  DAB7 : Subsystem  mask(Data Adquisition Board){filter=off, approx=Bessel, order=2, numerator=[], denominator=[], freq=180, resdis=off, vertres=12, xmax=10, winsize=40, G=1.0, fs=Freq*40}
      mask prompts: filter "Disable Analog Filter"; approx "Filter approximation"; numerator "Free expression filter: numerator(descending order of s)"; denominator "Free expression filter: denominator:"; freq "Cut-off frequency"; resdis "Disable Vertical Resolution"; vertres "Vertical Resolution: No. of bits"; xmax "Vertical Resolution: signal range"; winsize "Window size"; G "Gain"; fs "Sampling frequency"
      mask help: Performs analog filtering, signal conditioning and sampling. A single signal is the input, a buffer with the signal samples is the output. The options include analog filter enable/disable switch, type, order and cut-off frequency of the analog filter, conditioning gain, sampling frequency, number of bits, the length of the buffer.
      mask init:
      | dab1
      mask TypeOptions approx: Bessel | Tschebyscheff | Butterworth | free expression
      mask TypeOptions order: 2 | 3 | 4
      mask TypeOptions vertres: 8 | 12 | 16
      mask Display: disp('DAB')
  Degrees to Radians1 : simulink_extras/Transformations/Degrees to Radians
  Degrees to Radians2 : simulink_extras/Transformations/Degrees to Radians
  Degrees to Radians3 : simulink_extras/Transformations/Degrees to Radians
  Demux : Demux  Outputs=2
  Demux1 : Demux  Outputs=2
  Demux2 : Demux  Outputs=2
  Derivative : Derivative
  Derivative1 : Derivative
  Derivative2 : Derivative
  Magnitude-Angle to Complex : MagnitudeAngleToComplex
  Magnitude-Angle to Complex1 : MagnitudeAngleToComplex
  Magnitude-Angle to Complex2 : MagnitudeAngleToComplex
  Mux : Mux  Inputs=12
  Terminator : Terminator
  sum : Sum  Inputs=+--  SaturateOnIntegerOverflow=on  InputSameDT=on  OutDataTypeStr=Inherit: Same as first input
  Icomp : Outport  VectorParamsAs1DForOutWhenUnconnected=on
  wires:
  VA/1 -> Derivative2/1
  VC/1 -> Derivative/1
  " 5"/1 -> Demux2/1
  Demux1/2 -> Degrees to Radians2/1
  Demux1/1 -> Magnitude-Angle to Complex1/1
  " 7"/1 -> Demux/1
  Derivative1/1 -> DAB6/1(a)
  DAB6/1(d) -> " 6"/1
  " 6"/1 -> Demux1/1
  VB/1 -> Derivative1/1
  Mux/1 -> Terminator/1
  " 5"/5 -> Mux/4
  Derivative/1 -> DAB5/1(a)
  DAB5/1(d) -> " 5"/1
  Cpg/1 -> Compensating Current/1
  " 5"/2 -> Mux/1
  " 5"/3 -> Mux/2
  " 5"/4 -> Mux/3
  sum/1 -> Cpp/1
  Compensating Current/1 -> Icomp/1
  *2/1 -> sum/1
  Cpp/1 -> Compensating Current/2
  Derivative2/1 -> DAB7/1(a)
  DAB7/1(d) -> " 7"/1
  " 7"/2 -> Mux/9
  " 7"/3 -> Mux/10
  " 7"/4 -> Mux/11
  " 7"/5 -> Mux/12
  " 6"/2 -> Mux/5
  " 6"/3 -> Mux/6
  " 6"/4 -> Mux/7
  " 6"/5 -> Mux/8
  Demux2/1 -> Magnitude-Angle to Complex/1
  Magnitude-Angle to Complex/1 -> *2/1, Cpg/1
  Magnitude-Angle to Complex1/1 -> sum/2
  Demux/1 -> Magnitude-Angle to Complex2/1
  Magnitude-Angle to Complex2/1 -> sum/3
  Demux/2 -> Degrees to Radians1/1
  Degrees to Radians1/1 -> Magnitude-Angle to Complex2/2
  Degrees to Radians2/1 -> Magnitude-Angle to Complex1/2
  Demux2/2 -> Degrees to Radians3/1
  Degrees to Radians3/1 -> Magnitude-Angle to Complex/2

== system WindFarm_2023_BaseModel_v2/SM_WT1/Differential Element 2/Main Protection (Current Differential)/Current Differential Protection for Phase A ==
  Ilocal : Inport
  Iremote : Inport  Port=2
  Icomp : Inport  Port=3
  " " : elements/   fo=Freq  window_size=40  harmonic=[1 2 3 4 5]
  " 1" : elements/   fo=Freq  window_size=40  harmonic=[1 2 3 4 5]
  Comparing Current at Master Station : Sum  Inputs=+-  SaturateOnIntegerOverflow=on  InputSameDT=on  OutDataTypeStr=Inherit: Same as first input
  Comparision Scheme : Subsystem
  DAB4 : Subsystem  mask(Data Adquisition Board){filter=off, approx=Bessel, order=2, numerator=[], denominator=[], freq=180, resdis=off, vertres=12, xmax=10, winsize=40, G=1.0, fs=Freq*40}
      mask prompts: filter "Disable Analog Filter"; approx "Filter approximation"; numerator "Free expression filter: numerator(descending order of s)"; denominator "Free expression filter: denominator:"; freq "Cut-off frequency"; resdis "Disable Vertical Resolution"; vertres "Vertical Resolution: No. of bits"; xmax "Vertical Resolution: signal range"; winsize "Window size"; G "Gain"; fs "Sampling frequency"
      mask help: Performs analog filtering, signal conditioning and sampling. A single signal is the input, a buffer with the signal samples is the output. The options include analog filter enable/disable switch, type, order and cut-off frequency of the analog filter, conditioning gain, sampling frequency, number of bits, the length of the buffer.
      mask init:
      | dab1
      mask TypeOptions approx: Bessel | Tschebyscheff | Butterworth | free expression
      mask TypeOptions order: 2 | 3 | 4
      mask TypeOptions vertres: 8 | 12 | 16
      mask Display: disp('DAB')
  DAB8 : Subsystem  mask(Data Adquisition Board){filter=off, approx=Bessel, order=2, numerator=[], denominator=[], freq=180, resdis=off, vertres=12, xmax=10, winsize=40, G=1.0, fs=Freq*40}
      mask prompts: filter "Disable Analog Filter"; approx "Filter approximation"; numerator "Free expression filter: numerator(descending order of s)"; denominator "Free expression filter: denominator:"; freq "Cut-off frequency"; resdis "Disable Vertical Resolution"; vertres "Vertical Resolution: No. of bits"; xmax "Vertical Resolution: signal range"; winsize "Window size"; G "Gain"; fs "Sampling frequency"
      mask help: Performs analog filtering, signal conditioning and sampling. A single signal is the input, a buffer with the signal samples is the output. The options include analog filter enable/disable switch, type, order and cut-off frequency of the analog filter, conditioning gain, sampling frequency, number of bits, the length of the buffer.
      mask init:
      | dab1
      mask TypeOptions approx: Bessel | Tschebyscheff | Butterworth | free expression
      mask TypeOptions order: 2 | 3 | 4
      mask TypeOptions vertres: 8 | 12 | 16
      mask Display: disp('DAB')
  Degrees to Radians : simulink_extras/Transformations/Degrees to Radians
  Degrees to Radians1 : simulink_extras/Transformations/Degrees to Radians
  Demux1 : Demux  Outputs=2
  Demux2 : Demux  Outputs=2
  Gain : Gain  SaturateOnIntegerOverflow=on  OutDataTypeStr=Inherit: Same as input  ParamDataTypeStr=Inherit: Same as input
  Gain1 : Gain  SaturateOnIntegerOverflow=on  OutDataTypeStr=Inherit: Same as input  ParamDataTypeStr=Inherit: Same as input
  Magnitude-Angle to Complex : MagnitudeAngleToComplex
  Magnitude-Angle to Complex1 : MagnitudeAngleToComplex
  Mux1 : Mux
  Mux2 : Mux
  Terminator1 : Terminator
  Terminator2 : Terminator
  Trip : Outport  InitialOutput=0  VectorParamsAs1DForOutWhenUnconnected=on
  wires:
  Gain1/1 -> Comparing Current at Master Station/2
  " 1"/2 -> Mux2/1
  " 1"/4 -> Mux2/3
  " 1"/3 -> Mux2/2
  Mux2/1 -> Terminator2/1
  Gain/1 -> DAB8/1(a)
  Iremote/1 -> Gain/1
  " 1"/1 -> Demux2/1
  DAB8/1(d) -> " 1"/1
  Magnitude-Angle to Complex1/1 -> Comparision Scheme/2(I_Master)
  Demux2/2 -> Degrees to Radians/1
  Degrees to Radians/1 -> Magnitude-Angle to Complex1/2
  Demux2/1 -> Magnitude-Angle to Complex1/1
  " "/5 -> Mux1/4
  " "/4 -> Mux1/3
  " "/3 -> Mux1/2
  " "/2 -> Mux1/1
  Mux1/1 -> Terminator1/1
  " "/1 -> Demux1/1
  Comparision Scheme/1(Pickup) -> Trip/1
  DAB4/1(d) -> " "/1
  Ilocal/1 -> DAB4/1(a)
  Magnitude-Angle to Complex/1 -> Comparing Current at Master Station/1
  Icomp/1 -> Gain1/1
  Demux1/2 -> Degrees to Radians1/1
  Degrees to Radians1/1 -> Magnitude-Angle to Complex/2
  Comparing Current at Master Station/1 -> Comparision Scheme/1(I_Slave)
  " 1"/5 -> Mux2/4
  Demux1/1 -> Magnitude-Angle to Complex/1
